simulink model "HW6_switching"  (R2019a)
settings: Solver=VariableStepAuto  StartTime=0.0  StopTime=100  RelTol=1e-3
libraries: simulink x4
settings Model: Creator=morga  LastModifiedBy=morga

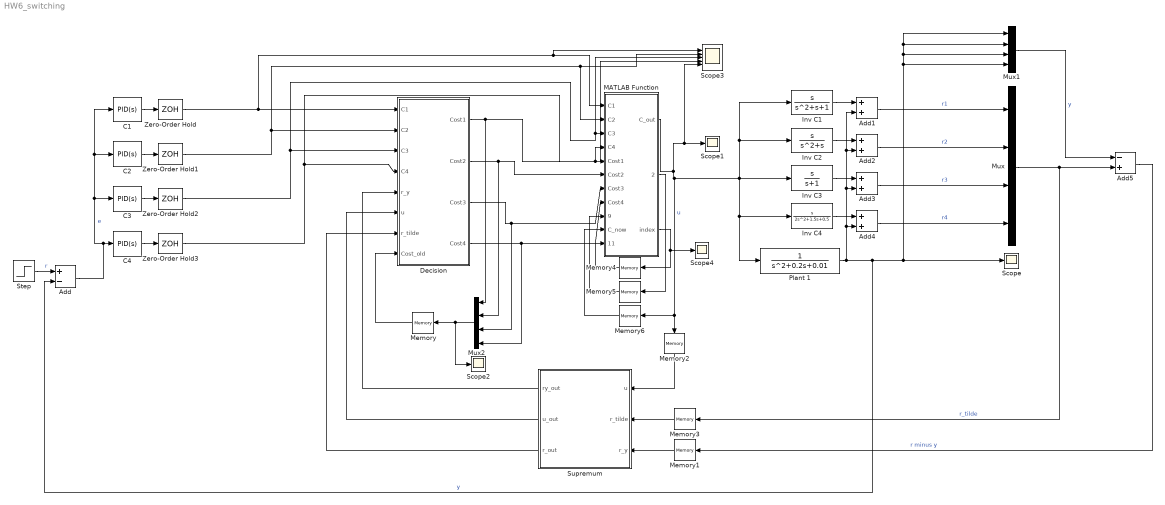
== system HW6_switching ==
  Add : Sum  Inputs=+-
  Add{1..4} (4 alike) : Sum
  Add5 : Sum  Inputs=-+
  C1 : simulink/Continuous/PID Controller  Controller=PID  Form=Parallel  TimeDomain=Continuous-time  SampleTime=0.1  IntegratorMethod=Forward Euler  FilterMethod=Forward Euler  ControllerParametersSource=internal  P=1  I=1  D=1  UseFilter=on  N=100  TunerSelectOption=Transfer Function Based (PID Tuner App)  InitialConditionSource=internal  InitialConditionForIntegrator=0  InitialConditionForFilter=0  DifferentiatorICPrevScaledInput=0  ExternalReset=none  TrackingMode=off  Kt=1  LimitOutput=off  UpperSaturationLimit=inf  LowerSaturationLimit=-inf  LinearizeAsGain=on  AntiWindupMode=none  Kb=1  POutMin=[]  POutMax=[]  IOutMin=[]  IOutMax=[]  DOutMin=[]  DOutMax=[]  NOutMin=[]  NOutMax=[]  SumOutMin=[]  SumOutMax=[]  SaturationOutMin=[]  SaturationOutMax=[]  PParamMin=[]  PParamMax=[]  IParamMin=[]  IParamMax=[]  DParamMin=[]  DParamMax=[]  NParamMin=[]  NParamMax=[]  KbParamMin=[]  KbParamMax=[]  KtParamMin=[]  KtParamMax=[]  KbOutMin=[]  KbOutMax=[]  KtOutMin=[]  KtOutMax=[]  IntegratorOutMin=[]  IntegratorOutMax=[]  FilterOutMin=[]  FilterOutMax=[]  SumI1OutMin=[]  SumI1OutMax=[]  SumI2OutMin=[]  SumI2OutMax=[]  SumI3OutMin=[]  SumI3OutMax=[]  SumI4OutMin=[]  SumI4OutMax=[]  SumDOutMin=[]  SumDOutMax=[]  DifferentiatorOutMin=[]  DifferentiatorOutMax=[]  FilterDiffOutCoefMin=[]  FilterDiffOutCoefMax=[]  ReciprocalOutMin=[]  ReciprocalOutMax=[]  SumDenOutMin=[]  SumDenOutMax=[]  SumNumOutMin=[]  SumNumOutMax=[]  DivideOutMin=[]  DivideOutMax=[]  IntegratorContinuousStateAttributes=''  IntegratorStateMustResolveToSignalObject=off  IntegratorRTWStateStorageClass=Auto  FilterContinuousStateAttributes=''  FilterStateMustResolveToSignalObject=off  FilterRTWStateStorageClass=Auto  ParallelPVariant=InternalParameters  IdealPVariant=Disabled  IVariant=InternalParameters  DVariant=InternalParameters  IntegratorVariant=Continuous  SatVariant=Disabled  AWVariant=Passthrough  PCopyVariant=Disabled  TRVariant=Disabled  FdbkBlocksVariant=Forward  IdealPFdbkVariant=Disabled  SatFdbkVariant=Disabled  DerivativeFilterVariant=ContFilter  NVariant=InternalParameters  NCopyVariant=Disabled  FilterICVariant=InternalICsFilter  IntegratorICVariant=InternalICs  ExternalResetVariant=Disabled  TRSumVariant=Passthrough  SumFdbkVariant=Disabled  SumVariant=Sum_PID
  C2 : simulink/Continuous/PID Controller  Controller=PID  Form=Parallel  TimeDomain=Continuous-time  SampleTime=0.1  IntegratorMethod=Forward Euler  FilterMethod=Forward Euler  ControllerParametersSource=internal  P=1  I=0  D=1  UseFilter=on  N=100  TunerSelectOption=Transfer Function Based (PID Tuner App)  InitialConditionSource=internal  InitialConditionForIntegrator=0  InitialConditionForFilter=0  DifferentiatorICPrevScaledInput=0  ExternalReset=none  TrackingMode=off  Kt=1  LimitOutput=off  UpperSaturationLimit=inf  LowerSaturationLimit=-inf  LinearizeAsGain=on  AntiWindupMode=none  Kb=1  POutMin=[]  POutMax=[]  IOutMin=[]  IOutMax=[]  DOutMin=[]  DOutMax=[]  NOutMin=[]  NOutMax=[]  SumOutMin=[]  SumOutMax=[]  SaturationOutMin=[]  SaturationOutMax=[]  PParamMin=[]  PParamMax=[]  IParamMin=[]  IParamMax=[]  DParamMin=[]  DParamMax=[]  NParamMin=[]  NParamMax=[]  KbParamMin=[]  KbParamMax=[]  KtParamMin=[]  KtParamMax=[]  KbOutMin=[]  KbOutMax=[]  KtOutMin=[]  KtOutMax=[]  IntegratorOutMin=[]  IntegratorOutMax=[]  FilterOutMin=[]  FilterOutMax=[]  SumI1OutMin=[]  SumI1OutMax=[]  SumI2OutMin=[]  SumI2OutMax=[]  SumI3OutMin=[]  SumI3OutMax=[]  SumI4OutMin=[]  SumI4OutMax=[]  SumDOutMin=[]  SumDOutMax=[]  DifferentiatorOutMin=[]  DifferentiatorOutMax=[]  FilterDiffOutCoefMin=[]  FilterDiffOutCoefMax=[]  ReciprocalOutMin=[]  ReciprocalOutMax=[]  SumDenOutMin=[]  SumDenOutMax=[]  SumNumOutMin=[]  SumNumOutMax=[]  DivideOutMin=[]  DivideOutMax=[]  IntegratorContinuousStateAttributes=''  IntegratorStateMustResolveToSignalObject=off  IntegratorRTWStateStorageClass=Auto  FilterContinuousStateAttributes=''  FilterStateMustResolveToSignalObject=off  FilterRTWStateStorageClass=Auto  ParallelPVariant=InternalParameters  IdealPVariant=Disabled  IVariant=InternalParameters  DVariant=InternalParameters  IntegratorVariant=Continuous  SatVariant=Disabled  AWVariant=Passthrough  PCopyVariant=Disabled  TRVariant=Disabled  FdbkBlocksVariant=Forward  IdealPFdbkVariant=Disabled  SatFdbkVariant=Disabled  DerivativeFilterVariant=ContFilter  NVariant=InternalParameters  NCopyVariant=Disabled  FilterICVariant=InternalICsFilter  IntegratorICVariant=InternalICs  ExternalResetVariant=Disabled  TRSumVariant=Passthrough  SumFdbkVariant=Disabled  SumVariant=Sum_PID
  C3 : simulink/Continuous/PID Controller  Controller=PID  Form=Parallel  TimeDomain=Continuous-time  SampleTime=0.1  IntegratorMethod=Forward Euler  FilterMethod=Forward Euler  ControllerParametersSource=internal  P=1  I=1  D=0  UseFilter=on  N=100  TunerSelectOption=Transfer Function Based (PID Tuner App)  InitialConditionSource=internal  InitialConditionForIntegrator=0  InitialConditionForFilter=0  DifferentiatorICPrevScaledInput=0  ExternalReset=none  TrackingMode=off  Kt=1  LimitOutput=off  UpperSaturationLimit=inf  LowerSaturationLimit=-inf  LinearizeAsGain=on  AntiWindupMode=none  Kb=1  POutMin=[]  POutMax=[]  IOutMin=[]  IOutMax=[]  DOutMin=[]  DOutMax=[]  NOutMin=[]  NOutMax=[]  SumOutMin=[]  SumOutMax=[]  SaturationOutMin=[]  SaturationOutMax=[]  PParamMin=[]  PParamMax=[]  IParamMin=[]  IParamMax=[]  DParamMin=[]  DParamMax=[]  NParamMin=[]  NParamMax=[]  KbParamMin=[]  KbParamMax=[]  KtParamMin=[]  KtParamMax=[]  KbOutMin=[]  KbOutMax=[]  KtOutMin=[]  KtOutMax=[]  IntegratorOutMin=[]  IntegratorOutMax=[]  FilterOutMin=[]  FilterOutMax=[]  SumI1OutMin=[]  SumI1OutMax=[]  SumI2OutMin=[]  SumI2OutMax=[]  SumI3OutMin=[]  SumI3OutMax=[]  SumI4OutMin=[]  SumI4OutMax=[]  SumDOutMin=[]  SumDOutMax=[]  DifferentiatorOutMin=[]  DifferentiatorOutMax=[]  FilterDiffOutCoefMin=[]  FilterDiffOutCoefMax=[]  ReciprocalOutMin=[]  ReciprocalOutMax=[]  SumDenOutMin=[]  SumDenOutMax=[]  SumNumOutMin=[]  SumNumOutMax=[]  DivideOutMin=[]  DivideOutMax=[]  IntegratorContinuousStateAttributes=''  IntegratorStateMustResolveToSignalObject=off  IntegratorRTWStateStorageClass=Auto  FilterContinuousStateAttributes=''  FilterStateMustResolveToSignalObject=off  FilterRTWStateStorageClass=Auto  ParallelPVariant=InternalParameters  IdealPVariant=Disabled  IVariant=InternalParameters  DVariant=InternalParameters  IntegratorVariant=Continuous  SatVariant=Disabled  AWVariant=Passthrough  PCopyVariant=Disabled  TRVariant=Disabled  FdbkBlocksVariant=Forward  IdealPFdbkVariant=Disabled  SatFdbkVariant=Disabled  DerivativeFilterVariant=ContFilter  NVariant=InternalParameters  NCopyVariant=Disabled  FilterICVariant=InternalICsFilter  IntegratorICVariant=InternalICs  ExternalResetVariant=Disabled  TRSumVariant=Passthrough  SumFdbkVariant=Disabled  SumVariant=Sum_PID
  C4 : simulink/Continuous/PID Controller  Controller=PID  Form=Parallel  TimeDomain=Continuous-time  SampleTime=0.1  IntegratorMethod=Forward Euler  FilterMethod=Forward Euler  ControllerParametersSource=internal  P=2  I=0.5  D=1.5  UseFilter=on  N=100  TunerSelectOption=Transfer Function Based (PID Tuner App)  InitialConditionSource=internal  InitialConditionForIntegrator=0  InitialConditionForFilter=0  DifferentiatorICPrevScaledInput=0  ExternalReset=none  TrackingMode=off  Kt=1  LimitOutput=off  UpperSaturationLimit=inf  LowerSaturationLimit=-inf  LinearizeAsGain=on  AntiWindupMode=none  Kb=1  POutMin=[]  POutMax=[]  IOutMin=[]  IOutMax=[]  DOutMin=[]  DOutMax=[]  NOutMin=[]  NOutMax=[]  SumOutMin=[]  SumOutMax=[]  SaturationOutMin=[]  SaturationOutMax=[]  PParamMin=[]  PParamMax=[]  IParamMin=[]  IParamMax=[]  DParamMin=[]  DParamMax=[]  NParamMin=[]  NParamMax=[]  KbParamMin=[]  KbParamMax=[]  KtParamMin=[]  KtParamMax=[]  KbOutMin=[]  KbOutMax=[]  KtOutMin=[]  KtOutMax=[]  IntegratorOutMin=[]  IntegratorOutMax=[]  FilterOutMin=[]  FilterOutMax=[]  SumI1OutMin=[]  SumI1OutMax=[]  SumI2OutMin=[]  SumI2OutMax=[]  SumI3OutMin=[]  SumI3OutMax=[]  SumI4OutMin=[]  SumI4OutMax=[]  SumDOutMin=[]  SumDOutMax=[]  DifferentiatorOutMin=[]  DifferentiatorOutMax=[]  FilterDiffOutCoefMin=[]  FilterDiffOutCoefMax=[]  ReciprocalOutMin=[]  ReciprocalOutMax=[]  SumDenOutMin=[]  SumDenOutMax=[]  SumNumOutMin=[]  SumNumOutMax=[]  DivideOutMin=[]  DivideOutMax=[]  IntegratorContinuousStateAttributes=''  IntegratorStateMustResolveToSignalObject=off  IntegratorRTWStateStorageClass=Auto  FilterContinuousStateAttributes=''  FilterStateMustResolveToSignalObject=off  FilterRTWStateStorageClass=Auto  ParallelPVariant=InternalParameters  IdealPVariant=Disabled  IVariant=InternalParameters  DVariant=InternalParameters  IntegratorVariant=Continuous  SatVariant=Disabled  AWVariant=Passthrough  PCopyVariant=Disabled  TRVariant=Disabled  FdbkBlocksVariant=Forward  IdealPFdbkVariant=Disabled  SatFdbkVariant=Disabled  DerivativeFilterVariant=ContFilter  NVariant=InternalParameters  NCopyVariant=Disabled  FilterICVariant=InternalICsFilter  IntegratorICVariant=InternalICs  ExternalResetVariant=Disabled  TRSumVariant=Passthrough  SumFdbkVariant=Disabled  SumVariant=Sum_PID
  Decision : MATLAB Function  TreatAsAtomicUnit=on
  Inv C1 : TransferFcn  Numerator=[1 0]  Denominator=[1 1 1]
  Inv C2 : TransferFcn  Numerator=[1 0]  Denominator=[1 1 0]
  Inv C3 : TransferFcn  Numerator=[1 0]  Denominator=[1 1]
  Inv C4 : TransferFcn  Numerator=[1 0]  Denominator=[2 1.5 0.5]
  MATLAB Function : MATLAB Function  TreatAsAtomicUnit=on
  Memory : Memory  InitialCondition=[0 0 0 0]  InheritSampleTime=on  LinearizeAsDelay=on
  Memory1 : Memory  InitialCondition=[0 0 0 0]
  Memory2 : Memory  InheritSampleTime=on
  Memory3 : Memory  InitialCondition=[0 0 0 0]
  Memory4 : Memory  InitialCondition=1  InheritSampleTime=on  LinearizeAsDelay=on
  Memory5 : Memory  InheritSampleTime=on  LinearizeAsDelay=on
  Memory6 : Memory  InheritSampleTime=on  LinearizeAsDelay=on
  Mux : Mux
  Mux1 : Mux
  Mux2 : Mux
  Plant 1 : TransferFcn  Denominator=[1 0.2 0.01]
  Scope{,1..2,4} (4 alike) : Scope
  Scope3 : Scope  NumInputPorts=5
  Step : Step  Time=0  SampleTime=0
  Supremum : Subsystem
  Zero-Order Hold{,1..3} (4 alike) : ZeroOrderHold  SampleTime=0.1
  wires:
  Plant 1/1 -> Mux1/1, Mux1/2, Mux1/3, Mux1/4, Scope/1, Add/2, Add1/2, Add2/2, Add3/2, Add4/2  "y"
  MATLAB Function/1(C_out) -> Memory6/1, Memory2/1, Plant 1/1, Inv C4/1, Inv C1/1, Inv C2/1, Inv C3/1, Scope3/5, Scope1/1  "u"
  Step/1 -> Add/1  "r"
  Add/1 -> C2/1, C1/1, C3/1, C4/1  "e"
  Inv C1/1 -> Add1/1
  Inv C2/1 -> Add2/1
  Inv C3/1 -> Add3/1
  Inv C4/1 -> Add4/1
  Add1/1 -> Mux/1  "r1"
  Add2/1 -> Mux/2  "r2"
  C3/1 -> Zero-Order Hold2/1
  C1/1 -> Zero-Order Hold/1
  C2/1 -> Zero-Order Hold1/1
  C4/1 -> Zero-Order Hold3/1
  Decision/1(Cost1) -> MATLAB Function/5(Cost1), Mux2/1
  Decision/2(Cost2) -> Mux2/2, MATLAB Function/6(Cost2)
  Decision/3(Cost3) -> Mux2/3, MATLAB Function/7(Cost3)
  Decision/4(Cost4) -> Mux2/4, MATLAB Function/8(Cost4)
  Add3/1 -> Mux/3  "r3"
  Add4/1 -> Mux/4  "r4"
  Mux/1 -> Add5/2, Memory3/1  "r_tilde"
  Supremum/1(ry_out) -> Decision/5(r_y)
  Supremum/2(u_out) -> Decision/6(u)
  Supremum/3(r_out) -> Decision/7(r_tilde)
  Mux1/1 -> Add5/1  "y"
  Add5/1 -> Memory1/1  "r minus y"
  Mux2/1 -> Memory/1, Scope2/1
  Memory/1 -> Decision/8(Cost_old)
  Memory1/1 -> Supremum/3(r_y)
  Memory2/1 -> Supremum/1(u)
  Memory3/1 -> Supremum/2(r_tilde)
  Zero-Order Hold/1 -> Decision/1(C1), Scope3/1, MATLAB Function/1(C1)
  Zero-Order Hold1/1 -> Decision/2(C2), MATLAB Function/2(C2), Scope3/2
  Zero-Order Hold2/1 -> Scope3/3, MATLAB Function/3(C3), Decision/3(C3)
  Zero-Order Hold3/1 -> Decision/4(C4), Scope3/4, MATLAB Function/4(C4)
  MATLAB Function/2(time_out) -> Memory5/1
  Memory5/1 -> MATLAB Function/9(time_count)
  Memory6/1 -> MATLAB Function/10(C_now)
  MATLAB Function/3(index) -> Scope4/1, Memory4/1
  Memory4/1 -> MATLAB Function/11(index_past)

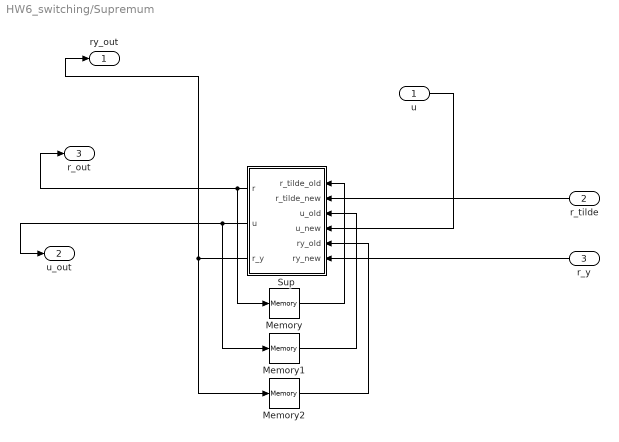
== system HW6_switching/Supremum ==
  u : Inport
  r_tilde : Inport  Port=2
  r_y : Inport  Port=3
  Memory : Memory  InitialCondition=[0 0 0 0]
  Memory1 : Memory
  Memory2 : Memory  InitialCondition=[0 0 0 0]
  Sup : MATLAB Function  TreatAsAtomicUnit=on
  ry_out : Outport  PortDimensions=4
  u_out : Outport  Port=2
  r_out : Outport  Port=3  PortDimensions=4
  wires:
  Sup/3(r_y) -> ry_out/1, Memory2/1
  Memory2/1 -> Sup/5(ry_old)
  Sup/1(r) -> r_out/1, Memory/1
  Sup/2(u) -> u_out/1, Memory1/1
  u/1 -> Sup/4(u_new)
  Memory1/1 -> Sup/3(u_old)
  r_tilde/1 -> Sup/2(r_tilde_new)
  Memory/1 -> Sup/1(r_tilde_old)
  r_y/1 -> Sup/6(ry_new)

== matlab function HW6_switching/Supremum/Sup ==
  data: r_tilde_old input; r_tilde_new input; u_old input; r output; u output; r_y output; u_new input; ry_old input; ry_new input
function [r, u, r_y] = fcn(r_tilde_old, r_tilde_new, u_old, u_new, ry_old, ry_new)

%% U
if abs(u_new) > abs(u_old)
    u = u_new;
else
    u = u_old;
end

%% Error
if abs(ry_old) > abs(ry_new)
    r_y = ry_old;
else
    r_y = ry_new;
end

%% R_tilde
if abs(r_tilde_old) > abs(r_tilde_new)
    r = r_tilde_old;
else
    r = r_tilde_new;
end

end

== matlab function HW6_switching/Decision ==
  data: C1 input; Cost1 output; C2 input; C3 input; C4 input; r_y input; u input; r_tilde input; Cost2 output; Cost3 output; Cost4 output; Cost_old input
function [Cost1, Cost2, Cost3, Cost4] = fcn(C1, C2, C3, C4, r_y, u, r_tilde, Cost_old)
% Make a decision of which controller should be used given situation
% Constants
a = 1;

input = [C1 C2 C3 C4];
Cost = zeros(4);
% Calculate the cost of each one
for i = 1:1:4
    Cost_update = (u^2 + r_y(i)^2) / (r_tilde(i)^2 + a);
    if Cost_update > Cost_old(i)
        Cost(i) = Cost_update;
    else
        Cost(i) = Cost_old(i);
    end
end
Cost1 = Cost(1);
Cost2 = Cost(2);
Cost3 = Cost(3);
Cost4 = Cost(4);
end

== matlab function HW6_switching/MATLAB Function ==
  data: C1 input; C_out output; C2 input; C3 input; C4 input; Cost1 input; Cost2 input; Cost3 input; Cost4 input; time_count input; C_now input; time_out output; index_past input; index output
function [C_out, time_out,index] = fcn(C1, C2, C3, C4, Cost1, Cost2, Cost3, Cost4, time_count, C_now, index_past)
C = [C1 C2 C3 C4];
dt = 0.1;
index = index_past; 

if time_count > 5
    Cost = [Cost1 Cost2 Cost3 Cost4];
    [maximum, index] = max(Cost);
    C_out = C(index);
else
    C_out = C_now;
end

if index == index_past
    time_out = time_count + dt;
else
    time_out = 0;
end

end
